simulink model "sum7"  (R2020b)
settings: Solver=VariableStepAuto  StartTime=0.0  StopTime=10.0  RelTol=1e-3
settings Model: Creator=Shivani  LastModifiedBy=Shivani

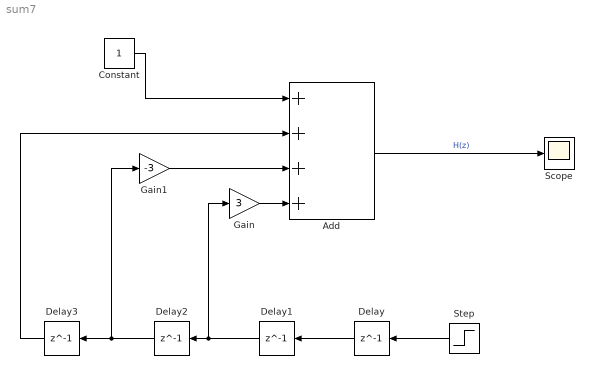
== system sum7 ==
  Add : Sum  Inputs=++++
  Constant : Constant
  Delay{,1..3} (4 alike) : Delay  DelayLength=1
  Gain : Gain  Gain=3
  Gain1 : Gain  Gain=-3
  Scope : Scope
  Step : Step  SampleTime=0
  wires:
  Add/1 -> Scope/1  "H(z)"
  Constant/1 -> Add/1
  Gain1/1 -> Add/3
  Step/1 -> Delay/1
  Delay/1 -> Delay1/1
  Delay1/1 -> Gain/1, Delay2/1
  Delay2/1 -> Gain1/1, Delay3/1
  Delay3/1 -> Add/2
  Gain/1 -> Add/4
